simulink model "carre"  (R2019a)
settings: Solver=VariableStepAuto  StartTime=0.0  StopTime=Tsim  RelTol=1e-3
values from neighbouring files (symbols this model uses):
  Te = 1/Fe    (= 3.125e-06)    [Laser.m]
undefined symbols (not defined in the file or in its folder): den
settings Model: Creator=vergnet  LastModifiedBy=vergnet

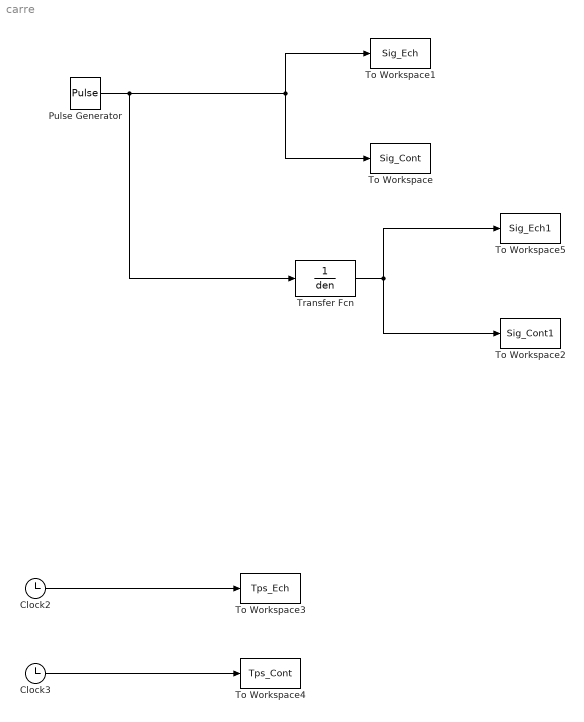
== system carre ==
  Clock2 : Clock
  Clock3 : Clock
  Pulse Generator : DiscretePulseGenerator  PulseType=Time based  Period=0.00001176470588235294  PulseWidth=50
  To Workspace : ToWorkspace  VariableName=Sig_Cont  SampleTime=Te/100
  To Workspace1 : ToWorkspace  VariableName=Sig_Ech  SampleTime=Te
  To Workspace2 : ToWorkspace  VariableName=Sig_Cont1  SampleTime=Te/100
  To Workspace3 : ToWorkspace  VariableName=Tps_Ech  SampleTime=Te
  To Workspace4 : ToWorkspace  VariableName=Tps_Cont  SampleTime=Te/100
  To Workspace5 : ToWorkspace  VariableName=Sig_Ech1  SampleTime=Te
  Transfer Fcn : TransferFcn  Denominator=den
  wires:
  Clock3/1 -> To Workspace4/1
  Clock2/1 -> To Workspace3/1
  Pulse Generator/1 -> Transfer Fcn/1, To Workspace1/1, To Workspace/1
  Transfer Fcn/1 -> To Workspace2/1, To Workspace5/1
